simulink model "subsys_ex"  (R2018a)
settings: Solver=VariableStepAuto  StartTime=0.0  StopTime=10.0  MaxStep=1e-3  RelTol=1e-3
settings Model: Creator=lenovo  LastModifiedBy=DELL

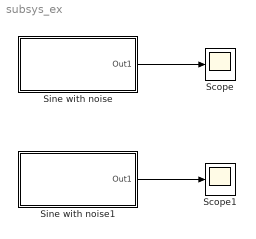
== system subsys_ex ==
  Scope : Scope
  Scope1 : Scope
  Sine with noise : Subsystem
  Sine with noise1 : Subsystem  mask(Sine with noise){s_a=1, s_f=1, n_m=0, n_v=0.1, m_a=plot}
      mask prompts: s_a "Sine Amplitude"; s_f "Sine Frequency"; n_m "Noise Mean"; n_v "Noise Variance"; m_a "Module appearance"
      mask help: The module is used to generate sinusoidal signals with normal random noise.
      mask TypeOptions m_a: string | image | plot
      mask Display:
      | ma=get_param(gcbh,'m_a');
      | if ma=="string"
      |     disp('Sine with noise');
      | elseif ma=="image"
      |     image(imread('Mask_demo01.jpg'));
      | elseif ma=="plot"
      |     sa=str2num(get_param(gcbh,'s_a'));
      |     sf=str2num(get_param(gcbh,'s_f'));
      |     nm=str2num(get_param(gcbh,'n_m'));
      |     nv=str2num(get_param(gcbh,'n_v'));
      |     T=2*pi/sf;
      |     t=0:T/100:2*T;
      |     s=rng(1);
      |     y=sa*sin(sf*t)+normrnd(nm,sqrt(nv),size(t));
      |     plot(t,y);
      | end
  wires:
  Sine with noise/1(Out1) -> Scope/1
  Sine with noise1/1(Out1) -> Scope1/1

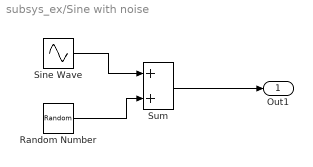
== system subsys_ex/Sine with noise ==
  Random Number : RandomNumber  Variance=0.1
  Sine Wave : Sin  SampleTime=0
  Sum : Sum
  Out1 : Outport  VectorParamsAs1DForOutWhenUnconnected=off
  wires:
  Random Number/1 -> Sum/2
  Sine Wave/1 -> Sum/1
  Sum/1 -> Out1/1

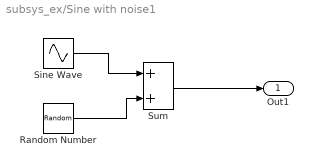
== system subsys_ex/Sine with noise1 ==
  Random Number : RandomNumber  Mean=n_m  Variance=n_v
  Sine Wave : Sin  Amplitude=s_a  Frequency=s_f  SampleTime=0
  Sum : Sum
  Out1 : Outport  VectorParamsAs1DForOutWhenUnconnected=off
  wires:
  Sum/1 -> Out1/1
  Sine Wave/1 -> Sum/1
  Random Number/1 -> Sum/2
